simulink library "PTOSim_Lib_org"  (R2014b)
settings: Solver=ode45  StartTime=0.0  StopTime=10.0  RelTol=1e-3
undefined symbols (not defined in the file or in its folder): accum, ddload, gen, machine, motor, pAeq, pAupper_limit, pBeq, pBupper_limit, piston, simu, tot, valve
libraries: PTOSim_Lib x10, WECSim_Lib x2
settings Model: RequirementInfo="{}  %GIDa_42666abb_d6d9_408c_ae24_f6520282b61c"  Creator=sor  LastModifiedBy=rso

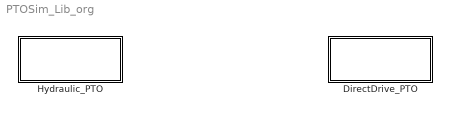
== system PTOSim_Lib_org ==
  DirectDrive_PTO : Subsystem  RequirementInfo="{}  %GIDa_5439fdb4_7c29_433c_8677_23bf92e18f11"
  Hydraulic_PTO : Subsystem  RequirementInfo={} %GIDa_f12a42eb_b9cb_4818_b573_b7dee4183a3b

== system PTOSim_Lib_org/DirectDrive_PTO ==
  Direct Drive PTO : Subsystem  mask{Parameter1=0}
      mask prompts: Parameter1 "pto"
  Electric Machine : Subsystem  RequirementInfo="{}  %GIDa_9a577bd3_d1cd_44c9_a605_4eaf21e33064"  mask{machine=machine}
      mask prompts: machine "Machine Name:"
  Load : Subsystem  mask(PTO-Sim Element){ddload=ddload}
      mask prompts: ddload "Load Name:"

== system PTOSim_Lib_org/Hydraulic_PTO ==
  Accumulator : Subsystem  mask(PTO-Sim Element){accum=accum}
      mask prompts: accum "Accumulator Name:"
  Generator : Subsystem  RequirementInfo="{}  %GIDa_30368e1c_dc2a_4605_bb50_ff3a423f2df5"  mask{gen=gen}
      mask prompts: gen "Generator Name"
  "High Accumulator " : Subsystem  mask(PTO-Sim Element){accum=accum}
      mask prompts: accum "Accumulator Name:"
  Hydraulic PTO : Subsystem  RequirementInfo="{}  %GIDa_b8f519ee_1776_4469_9852_74bfa511eadd"  mask{Parameter1=0}
      mask prompts: Parameter1 "pto"
  Low Accumulator : Subsystem  mask(PTO-Sim Element){accum=accum}
      mask prompts: accum "Accumulator"
  "Motor " : Subsystem  mask{motor=motor}
      mask prompts: motor "Motor Name:"
  "Piston " : Subsystem  RequirementInfo="{}  %GIDa_b30889e8_4129_48f7_be7d_bc9428e6e267"  mask(PTO-Sim Element){piston=piston}
      mask prompts: piston "Piston Name:"
  PistonX : Subsystem  mask{piston=piston}
      mask prompts: piston "Piston X Name:"
  Rectifiying Check Valve : Subsystem  RequirementInfo="{}  %GIDa_a75844df_5079_4f47_95bd_8083cdfec0d7"  mask{valve=valve}
      mask prompts: valve "Valve Name:"

== system PTOSim_Lib_org/DirectDrive_PTO/Direct Drive PTO ==
  vel : Inport
  Electric Machine : PTOSim_Lib/DirectDrive_PTO/Electric Machine  machine=machine
  Load : PTOSim_Lib/DirectDrive_PTO/Load  ddload=ddload
  Terminator1 : Terminator
  force : Outport
  wires:
  Electric Machine/2 -> Load/1
  Load/1 -> Electric Machine/2
  Electric Machine/1 -> force/1
  Load/2 -> Terminator1/1
  vel/1 -> Electric Machine/1

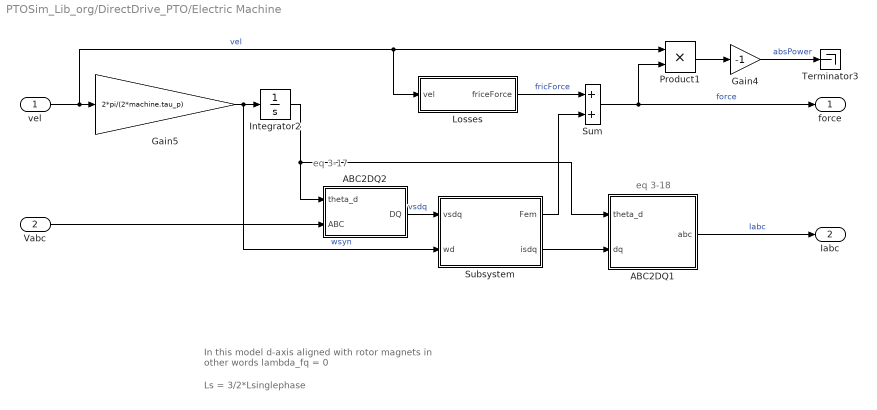
== system PTOSim_Lib_org/DirectDrive_PTO/Electric Machine ==
  note: In this model d-axis aligned with rotor magnets
      | in other words lambda_fq = 0
  note: Ls = 3/2*Lsinglephase
  note: eq 3-17
  note: eq 3-18
  vel : Inport
  Vabc : Inport  Port=2
  ABC2DQ1 : Subsystem
  ABC2DQ2 : Subsystem
  Gain4 : Gain  Gain=-1
  Gain5 : Gain  Gain=2*pi/(2*machine.tau_p)
  Integrator2 : Integrator  InitialCondition=machine.theta_d_0
  Losses : Subsystem
  Product1 : Product
  Subsystem : Subsystem
  Sum : Sum
  Terminator3 : Terminator
  force : Outport
  Iabc : Outport  Port=2
  wires:
  ABC2DQ2/1(DQ) -> Subsystem/1(vsdq)  "vsdq"
  ABC2DQ1/1(abc) -> Iabc/1  "Iabc"
  vel/1 -> Gain5/1, Losses/1(vel), Product1/1  "vel"
  Gain5/1 -> Subsystem/2(wd), Integrator2/1  "wsyn"
  Integrator2/1 -> ABC2DQ2/1(theta_d), ABC2DQ1/1(theta_d)
  Product1/1 -> Gain4/1
  Gain4/1 -> Terminator3/1  "absPower"
  Subsystem/1(Fem) -> Sum/2
  Vabc/1 -> ABC2DQ2/2(ABC)
  Subsystem/2(isdq) -> ABC2DQ1/2(dq)
  Losses/1(friceForce) -> Sum/1  "fricForce"
  Sum/1 -> Product1/2, force/1  "force"

== system PTOSim_Lib_org/DirectDrive_PTO/Load ==
  Iabc : Inport
  Gain : Gain  Gain=-1
  Gain1 : Gain  Gain=ddload.Rload
  Product : Product
  Sum of Elements : Sum  Inputs=+
  Vabc : Outport
  elecPower : Outport  Port=2
  wires:
  Gain/1 -> elecPower/1  "elecPower"
  Gain1/1 -> Product/1, Vabc/1  "Vabc"
  Product/1 -> Sum of Elements/1
  Iabc/1 -> Gain1/1, Product/2
  Sum of Elements/1 -> Gain/1

== system PTOSim_Lib_org/Hydraulic_PTO/Accumulator ==
  volFlowAccum : Inport
  volFlowM : Inport  Port=2
  Constant : Constant
  Constant3 : Constant  Value=accum.pIprecharge
  Constant4 : Constant  Value=accum.VI0
  Divide : Product  Inputs=*/
  Divide1 : Product  Inputs=*/
  Exponent : Constant  Value=1.4
  Integrator4 : Integrator  InitialCondition=accum.VIeq
  Math Function : Math  Operator=pow  SaturateOnIntegerOverflow=on
  Sum : Sum  Inputs=-+
  Sum2 : Sum
  pressure : Outport
  wires:
  Sum2/1 -> Integrator4/1  "volFlowAccum"
  Integrator4/1 -> Divide/1  "volAccum"
  Constant4/1 -> Divide/2
  Constant/1 -> Sum/2
  Divide/1 -> Sum/1
  Exponent/1 -> Math Function/2
  Sum/1 -> Math Function/1
  Math Function/1 -> Divide1/2
  Constant3/1 -> Divide1/1  "pI0"
  Divide1/1 -> pressure/1
  volFlowAccum/1 -> Sum2/1
  volFlowM/1 -> Sum2/2

== system PTOSim_Lib_org/Hydraulic_PTO/Generator ==
  torque : Inport
  omega : Inport  Port=2
  Base Motor Torque : Gain  Gain=-1/gen.TgenBase
  Base Motor Torque1 : Gain  Gain=1/gen.omegaBase
  Base Motor Torque2 : Gain  Gain=gen.driveEff
  Base Motor Torque3 : Gain  Gain=1/100
  PM p.u. Efficiency Lookup Table : Lookup_n-D  BreakpointsForDimension1=tot.Tpu(:,1)  BreakpointsForDimension2=tot.omegapu(1,:)  Table=tot.eff  InterpMethod=Flat  InputSameDT=on
  Product : Product  RndMeth=Zero
  Product1 : Product  RndMeth=Zero
  elecPower : Outport
  wires:
  Base Motor Torque2/1 -> elecPower/1  "elecPower"
  Product1/1 -> Base Motor Torque2/1
  Product/1 -> Product1/1  "genPower"
  Base Motor Torque3/1 -> Product1/2  "genEff"
  PM p.u. Efficiency Lookup Table/1 -> Base Motor Torque3/1
  omega/1 -> Product/2, Base Motor Torque1/1
  Base Motor Torque1/1 -> PM p.u. Efficiency Lookup Table/2  "omegaPU"
  torque/1 -> Base Motor Torque/1, Product/1
  Base Motor Torque/1 -> PM p.u. Efficiency Lookup Table/1  "torquePU"

== system PTOSim_Lib_org/Hydraulic_PTO/High Accumulator  ==
  volFlowHigh : Inport
  volFlowM : Inport  Port=2
  Constant : Constant
  Constant3 : Constant  Value=accum.pCprecharge
  Constant4 : Constant  Value=accum.VC0
  Divide : Product  Inputs=*/
  Divide1 : Product  Inputs=*/
  Exponent : Constant  Value=1.4
  Integrator4 : Integrator  InitialCondition=accum.VCeq
  Math Function : Math  Operator=pow  SaturateOnIntegerOverflow=on
  Sum : Sum  Inputs=-+
  Sum2 : Sum
  pressure : Outport
  wires:
  Sum2/1 -> Integrator4/1  "volFlowC"
  Integrator4/1 -> Divide/1  "volC"
  Constant4/1 -> Divide/2
  Constant/1 -> Sum/2
  Divide/1 -> Sum/1
  Exponent/1 -> Math Function/2
  Sum/1 -> Math Function/1
  Math Function/1 -> Divide1/2
  Constant3/1 -> Divide1/1  "pC0"
  Divide1/1 -> pressure/1
  volFlowHigh/1 -> Sum2/1
  volFlowM/1 -> Sum2/2

== system PTOSim_Lib_org/Hydraulic_PTO/Hydraulic PTO ==
  pos : Inport
  vel : Inport  Port=2
  Accumulator : PTOSim_Lib/Hydraulic_PTO/Accumulator  accum=highAccum
  Accumulator1 : PTOSim_Lib/Hydraulic_PTO/Accumulator  accum=lowAccum
  Generator : PTOSim_Lib/Hydraulic_PTO/Generator  gen=gen
  "Motor " : PTOSim_Lib/Hydraulic_PTO/Motor   motor=motor
  "Piston " : PTOSim_Lib/Hydraulic_PTO/Piston    piston=piston
  Rectifiying Check Valve : PTOSim_Lib/Hydraulic_PTO/Rectifiying  Check Valve  valve=valve
  Terminator : Terminator
  force : Outport
  wires:
  pos/1 -> "Piston "/1  "pos"
  vel/1 -> "Piston "/2  "vel"
  "Piston "/2 -> Rectifiying Check Valve/1  "topPressure"
  "Piston "/3 -> Rectifiying Check Valve/2  "bottomPressure"
  "Motor "/1 -> Generator/1
  "Motor "/2 -> Generator/2
  Accumulator/1 -> "Motor "/1, Rectifiying Check Valve/3  "highPressure"
  Accumulator1/1 -> Rectifiying Check Valve/4, "Motor "/2  "lowPressure"
  Generator/1 -> Terminator/1
  "Piston "/1 -> force/1
  Rectifiying Check Valve/1 -> "Piston "/3
  Rectifiying Check Valve/2 -> "Piston "/4
  Rectifiying Check Valve/3 -> Accumulator/1
  Rectifiying Check Valve/4 -> Accumulator1/1
  "Motor "/4 -> Accumulator1/2
  "Motor "/3 -> Accumulator/2

== system PTOSim_Lib_org/Hydraulic_PTO/Low Accumulator ==
  volFlowLow : Inport
  volFlowM : Inport  Port=2
  Constant : Constant
  Constant3 : Constant  Value=accum.pDprecharge
  Constant4 : Constant  Value=accum.VD0
  Divide : Product  Inputs=*/
  Divide1 : Product  Inputs=*/
  Exponent : Constant  Value=1.4
  Integrator4 : Integrator  InitialCondition=accum.VDeq
  Math Function : Math  Operator=pow  SaturateOnIntegerOverflow=on
  Sum : Sum  Inputs=-+
  Sum2 : Sum
  pressure : Outport
  wires:
  Sum2/1 -> Integrator4/1  "volFlowD"
  Integrator4/1 -> Divide/1  "volD"
  Constant4/1 -> Divide/2
  Constant/1 -> Sum/2
  Divide/1 -> Sum/1
  Exponent/1 -> Math Function/2
  Sum/1 -> Math Function/1
  Math Function/1 -> Divide1/2
  Constant3/1 -> Divide1/1  "pD0"
  Divide1/1 -> pressure/1
  volFlowLow/1 -> Sum2/1
  volFlowM/1 -> Sum2/2

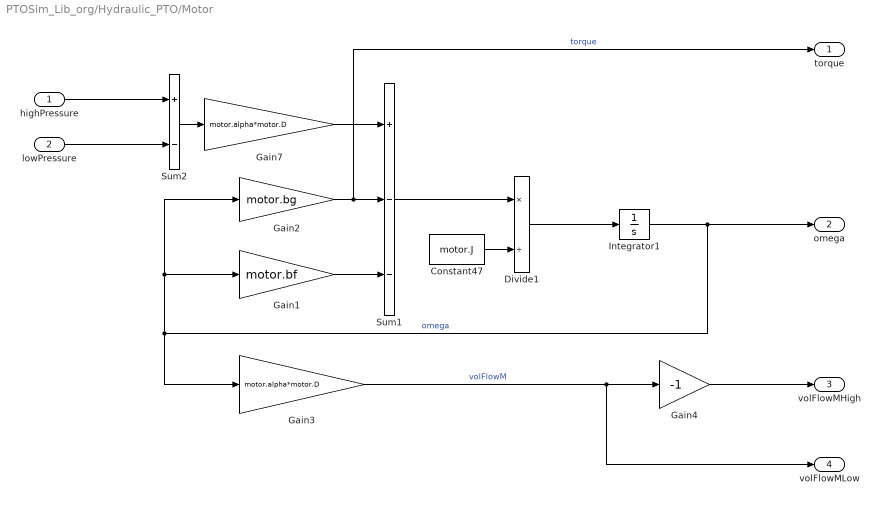
== system PTOSim_Lib_org/Hydraulic_PTO/Motor  ==
  highPressure : Inport
  lowPressure : Inport  Port=2
  Constant47 : Constant  Value=motor.J
  Divide1 : Product  Inputs=*/
  Gain1 : Gain  Gain=motor.bf
  Gain2 : Gain  Gain=motor.bg
  Gain3 : Gain  Gain=motor.alpha*motor.D
  Gain4 : Gain  Gain=-1
  Gain7 : Gain  Gain=motor.alpha*motor.D
  Integrator1 : Integrator  InitialCondition=motor.omegaInit
  Sum1 : Sum  Inputs=+--
  Sum2 : Sum  Inputs=+-
  torque : Outport
  omega : Outport  Port=2
  volFlowMHigh : Outport  Port=3
  volFlowMLow : Outport  Port=4
  wires:
  Gain7/1 -> Sum1/1
  Gain2/1 -> torque/1, Sum1/2  "torque"
  Gain1/1 -> Sum1/3
  Sum1/1 -> Divide1/1
  Constant47/1 -> Divide1/2
  Divide1/1 -> Integrator1/1
  Integrator1/1 -> omega/1, Gain3/1, Gain2/1, Gain1/1  "omega"
  Gain3/1 -> volFlowMLow/1, Gain4/1  "volFlowM"
  highPressure/1 -> Sum2/1
  lowPressure/1 -> Sum2/2
  Sum2/1 -> Gain7/1
  Gain4/1 -> volFlowMHigh/1

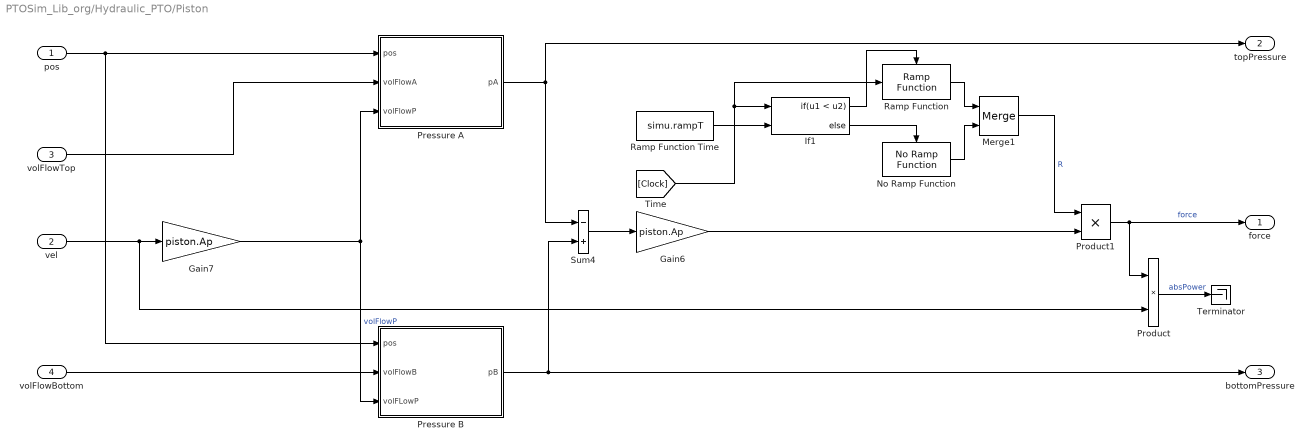
== system PTOSim_Lib_org/Hydraulic_PTO/Piston  ==
  pos : Inport
  vel : Inport  Port=2
  volFlowTop : Inport  Port=3
  volFlowBottom : Inport  Port=4
  Gain6 : Gain  Gain=piston.Ap
  Gain7 : Gain  Gain=piston.Ap
  If1 : If  NumInputs=2  IfExpression=u1 < u2
  Merge1 : Merge
  No Ramp Function : WECSim_Lib/Body Elements/Rigid Body/Wave Diffraction and Excitation Force Calculation/No Ramp Function
  Pressure A : Subsystem
  Pressure B : Subsystem  RequirementInfo="{}  %GIDa_18ee15fe_6148_4b69_b054_be19d4b47378"
  Product : Product
  Product1 : Product
  Ramp Function : WECSim_Lib/Body Elements/Rigid Body/Wave Diffraction and Excitation Force Calculation/Ramp Function
  Ramp Function Time : Constant  Value=simu.rampT
  Sum4 : Sum  Inputs=-+
  Terminator : Terminator
  force : Outport
  topPressure : Outport  Port=2
  bottomPressure : Outport  Port=3
  wires:
  Pressure A/1(pA) -> Sum4/1, topPressure/1
  Pressure B/1(pB) -> Sum4/2, bottomPressure/1
  Gain7/1 -> Pressure B/3(volFLowP), Pressure A/3(volFlowP)  "volFlowP"
  Product/1 -> Terminator/1  "absPower"
  pos/1 -> Pressure B/1(pos), Pressure A/1(pos)
  vel/1 -> Product/2, Gain7/1
  Sum4/1 -> Gain6/1
  [Clock] -> If1/1, Ramp Function/1
  Merge1/1 -> Product1/1  "R"
  Ramp Function Time/1 -> If1/2
  If1/2 -> No Ramp Function/Action
  If1/1 -> Ramp Function/Action
  Ramp Function/1 -> Merge1/1
  No Ramp Function/1 -> Merge1/2
  Gain6/1 -> Product1/2
  Product1/1 -> force/1, Product/1  "force"
  volFlowTop/1 -> Pressure A/2(volFlowA)
  volFlowBottom/1 -> Pressure B/2(volFlowB)

== system PTOSim_Lib_org/Hydraulic_PTO/PistonX ==
  pos : Inport
  vel : Inport  Port=2
  volFlowTop : Inport  Port=3
  volFlowBottom : Inport  Port=4
  Gain6 : Gain  Gain=piston.Ap
  Gain7 : Gain  Gain=piston.Ap
  Pressure A : PTOSim_Lib/Hydraulic_PTO/Piston  /Pressure A
  Pressure B : PTOSim_Lib/Hydraulic_PTO/Piston  /Pressure B
  Product : Product
  Sum4 : Sum  Inputs=-+
  Terminator : Terminator
  force : Outport
  topPressure : Outport  Port=2
  bottomPressure : Outport  Port=3
  wires:
  Pressure A/1 -> Sum4/1, topPressure/1
  Pressure B/1 -> Sum4/2, bottomPressure/1
  Gain7/1 -> Pressure B/3, Pressure A/3  "volFlowP"
  Product/1 -> Terminator/1  "absPower"
  pos/1 -> Pressure B/1, Pressure A/1
  vel/1 -> Product/2, Gain7/1
  Sum4/1 -> Gain6/1
  Gain6/1 -> force/1, Product/1  "force"
  volFlowTop/1 -> Pressure A/2
  volFlowBottom/1 -> Pressure B/2

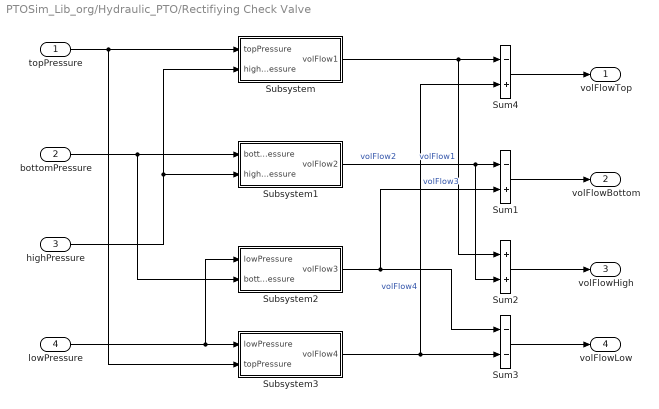
== system PTOSim_Lib_org/Hydraulic_PTO/Rectifiying Check Valve ==
  topPressure : Inport
  bottomPressure : Inport  Port=2
  highPressure : Inport  Port=3
  lowPressure : Inport  Port=4
  Subsystem : Subsystem  RequirementInfo="{}  %GIDa_43e7490a_26e5_4c96_a755_05599e7ab58d"
  Subsystem1 : Subsystem
  Subsystem2 : Subsystem
  Subsystem3 : Subsystem  RequirementInfo="{}  %GIDa_1d14c02d_1c58_4958_a821_20fe782ea22d"
  Sum1 : Sum  Inputs=-+
  Sum2 : Sum
  Sum3 : Sum  Inputs=--
  Sum4 : Sum  Inputs=-+
  volFlowTop : Outport
  volFlowBottom : Outport  Port=2
  volFlowHigh : Outport  Port=3
  volFlowLow : Outport  Port=4
  wires:
  topPressure/1 -> Subsystem3/2(topPressure), Subsystem/1(topPressure)
  bottomPressure/1 -> Subsystem2/2(bottomPressure), Subsystem1/1(bottomPressure)
  highPressure/1 -> Subsystem1/2(highPressure), Subsystem/2(highPressure)
  lowPressure/1 -> Subsystem2/1(lowPressure), Subsystem3/1(lowPressure)
  Subsystem3/1(volFlow4) -> Sum4/2, Sum3/2  "volFlow4"
  Subsystem2/1(volFlow3) -> Sum3/1, Sum1/2  "volFlow3"
  Subsystem1/1(volFlow2) -> Sum2/2, Sum1/1  "volFlow2"
  Subsystem/1(volFlow1) -> Sum2/1, Sum4/1  "volFlow1"
  Sum4/1 -> volFlowTop/1
  Sum1/1 -> volFlowBottom/1
  Sum2/1 -> volFlowHigh/1
  Sum3/1 -> volFlowLow/1

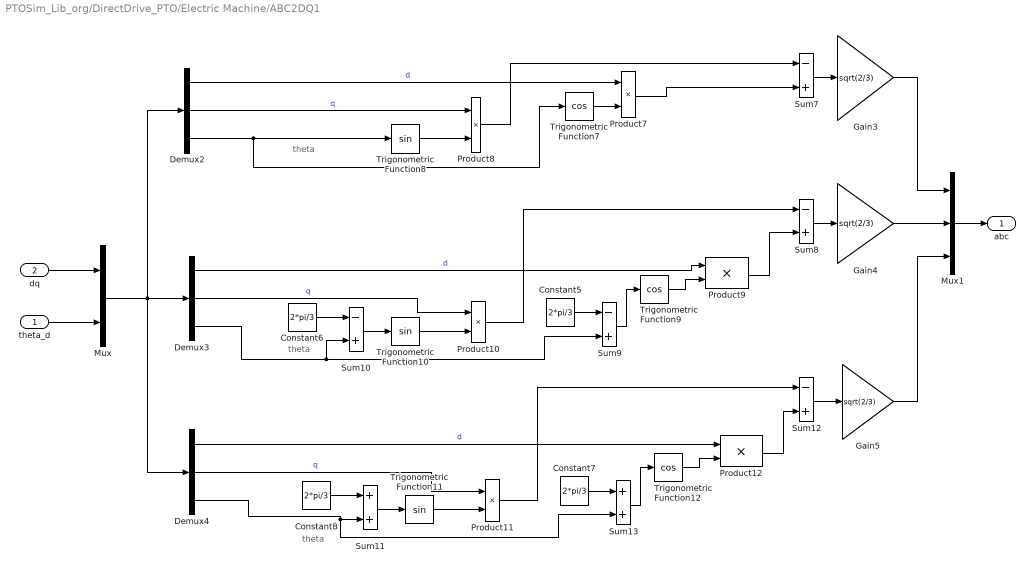
== system PTOSim_Lib_org/DirectDrive_PTO/Electric Machine/ABC2DQ1 ==
  note: theta
  note: theta
  note: theta
  theta_d : Inport
  dq : Inport  Port=2
  Constant{5..8} (4 alike) : Constant  Value=2*pi/3
  Demux2 : Demux  Outputs=3
  Demux3 : Demux  Outputs=3
  Demux4 : Demux  Outputs=3
  Gain3 : Gain  Gain=sqrt(2/3)  SaturateOnIntegerOverflow=on  OutDataTypeStr=Inherit: Same as input  ParamDataTypeStr=Inherit: Same as input
  Gain4 : Gain  Gain=sqrt(2/3)  SaturateOnIntegerOverflow=on  OutDataTypeStr=Inherit: Same as input  ParamDataTypeStr=Inherit: Same as input
  Gain5 : Gain  Gain=sqrt(2/3)  SaturateOnIntegerOverflow=on  OutDataTypeStr=Inherit: Same as input  ParamDataTypeStr=Inherit: Same as input
  Mux : Mux  Inputs=2
  Mux1 : Mux  Inputs=3
  Product{7..12} (6 alike) : Product  SaturateOnIntegerOverflow=on  InputSameDT=on  OutDataTypeStr=Inherit: Same as first input
  Sum{7..10,12} (5 alike) : Sum  Inputs=-+  SaturateOnIntegerOverflow=on  InputSameDT=on  OutDataTypeStr=Inherit: Same as first input
  Sum11 : Sum  SaturateOnIntegerOverflow=on  InputSameDT=on  OutDataTypeStr=Inherit: Same as first input
  Sum13 : Sum  SaturateOnIntegerOverflow=on  InputSameDT=on  OutDataTypeStr=Inherit: Same as first input
  Trigonometric Function10 : Trigonometry
  Trigonometric Function11 : Trigonometry
  Trigonometric Function12 : Trigonometry  Operator=cos
  Trigonometric Function7 : Trigonometry  Operator=cos
  Trigonometric Function8 : Trigonometry
  Trigonometric Function9 : Trigonometry  Operator=cos
  abc : Outport
  wires:
  Mux1/1 -> abc/1
  dq/1 -> Mux/1
  theta_d/1 -> Mux/2
  Mux/1 -> Demux4/1, Demux2/1, Demux3/1
  Trigonometric Function7/1 -> Product7/2
  Demux2/1 -> Product7/1  "d"
  Product7/1 -> Sum7/2
  Product8/1 -> Sum7/1
  Demux2/3 -> Trigonometric Function8/1, Trigonometric Function7/1
  Demux2/2 -> Product8/1  "q"
  Trigonometric Function9/1 -> Product9/2
  Demux3/1 -> Product9/1  "d"
  Product9/1 -> Sum8/2
  Product10/1 -> Sum8/1
  Demux3/3 -> Sum10/2, Sum9/2
  Trigonometric Function10/1 -> Product10/2
  Demux3/2 -> Product10/1  "q"
  Sum9/1 -> Trigonometric Function9/1
  Constant5/1 -> Sum9/1
  Sum10/1 -> Trigonometric Function10/1
  Constant6/1 -> Sum10/1
  Trigonometric Function12/1 -> Product12/2
  Demux4/1 -> Product12/1  "d"
  Product12/1 -> Sum12/2
  Product11/1 -> Sum12/1
  Demux4/3 -> Sum13/2, Sum11/2
  Trigonometric Function11/1 -> Product11/2
  Demux4/2 -> Product11/1  "q"
  Sum13/1 -> Trigonometric Function12/1
  Constant7/1 -> Sum13/1
  Sum11/1 -> Trigonometric Function11/1
  Constant8/1 -> Sum11/1
  Sum7/1 -> Gain3/1
  Sum8/1 -> Gain4/1
  Sum12/1 -> Gain5/1
  Gain3/1 -> Mux1/1
  Gain4/1 -> Mux1/2
  Gain5/1 -> Mux1/3
  Trigonometric Function8/1 -> Product8/2

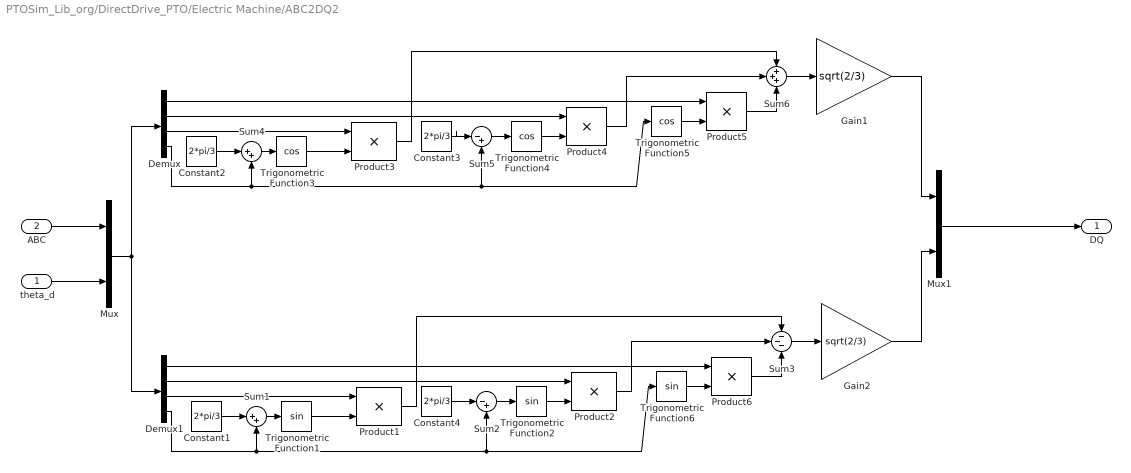
== system PTOSim_Lib_org/DirectDrive_PTO/Electric Machine/ABC2DQ2 ==
  theta_d : Inport
  ABC : Inport  Port=2
  Constant{1..4} (4 alike) : Constant  Value=2*pi/3
  Demux : Demux
  Demux1 : Demux
  Gain1 : Gain  Gain=sqrt(2/3)  SaturateOnIntegerOverflow=on  OutDataTypeStr=Inherit: Same as input  ParamDataTypeStr=Inherit: Same as input
  Gain2 : Gain  Gain=sqrt(2/3)  SaturateOnIntegerOverflow=on  OutDataTypeStr=Inherit: Same as input  ParamDataTypeStr=Inherit: Same as input
  Mux : Mux  Inputs=2
  Mux1 : Mux  Inputs=2
  Product{1..6} (6 alike) : Product  SaturateOnIntegerOverflow=on  InputSameDT=on  OutDataTypeStr=Inherit: Same as first input
  Sum1 : Sum  Inputs=|++  SaturateOnIntegerOverflow=on  InputSameDT=on  OutDataTypeStr=Inherit: Same as first input
  Sum2 : Sum  Inputs=|-+  SaturateOnIntegerOverflow=on  InputSameDT=on  OutDataTypeStr=Inherit: Same as first input
  Sum3 : Sum  Inputs=---  SaturateOnIntegerOverflow=on  InputSameDT=on  OutDataTypeStr=Inherit: Same as first input
  Sum4 : Sum  Inputs=|++  SaturateOnIntegerOverflow=on  InputSameDT=on  OutDataTypeStr=Inherit: Same as first input
  Sum5 : Sum  Inputs=|-+  SaturateOnIntegerOverflow=on  InputSameDT=on  OutDataTypeStr=Inherit: Same as first input
  Sum6 : Sum  Inputs=+++  SaturateOnIntegerOverflow=on  InputSameDT=on  OutDataTypeStr=Inherit: Same as first input
  Trigonometric Function1 : Trigonometry
  Trigonometric Function2 : Trigonometry
  Trigonometric Function3 : Trigonometry  Operator=cos
  Trigonometric Function4 : Trigonometry  Operator=cos
  Trigonometric Function5 : Trigonometry  Operator=cos
  Trigonometric Function6 : Trigonometry
  DQ : Outport
  wires:
  Mux1/1 -> DQ/1
  Product5/1 -> Sum6/3
  Constant2/1 -> Sum4/1
  Sum5/1 -> Trigonometric Function4/1
  Trigonometric Function4/1 -> Product4/2
  Trigonometric Function5/1 -> Product5/2
  Constant3/1 -> Sum5/1
  Sum6/1 -> Gain1/1
  Product3/1 -> Sum6/1
  Product4/1 -> Sum6/2
  Trigonometric Function3/1 -> Product3/2
  Gain1/1 -> Mux1/1
  ABC/1 -> Mux/1
  theta_d/1 -> Mux/2
  Demux/1 -> Product5/1
  Demux/2 -> Product4/1
  Demux/3 -> Product3/1
  Demux/4 -> Sum5/2, Trigonometric Function5/1, Sum4/2
  Mux/1 -> Demux/1, Demux1/1
  Sum4/1 -> Trigonometric Function3/1
  Product6/1 -> Sum3/3
  Constant1/1 -> Sum1/1
  Sum2/1 -> Trigonometric Function2/1
  Trigonometric Function2/1 -> Product2/2
  Trigonometric Function6/1 -> Product6/2
  Constant4/1 -> Sum2/1
  Sum3/1 -> Gain2/1
  Product1/1 -> Sum3/1
  Product2/1 -> Sum3/2
  Trigonometric Function1/1 -> Product1/2
  Gain2/1 -> Mux1/2
  Demux1/1 -> Product6/1
  Demux1/2 -> Product2/1
  Demux1/3 -> Product1/1
  Demux1/4 -> Sum1/2, Trigonometric Function6/1, Sum2/2
  Sum1/1 -> Trigonometric Function1/1

== system PTOSim_Lib_org/DirectDrive_PTO/Electric Machine/Losses ==
  vel : Inport
  Gain : Gain  Gain=machine.Bfric
  friceForce : Outport
  wires:
  vel/1 -> Gain/1
  Gain/1 -> friceForce/1

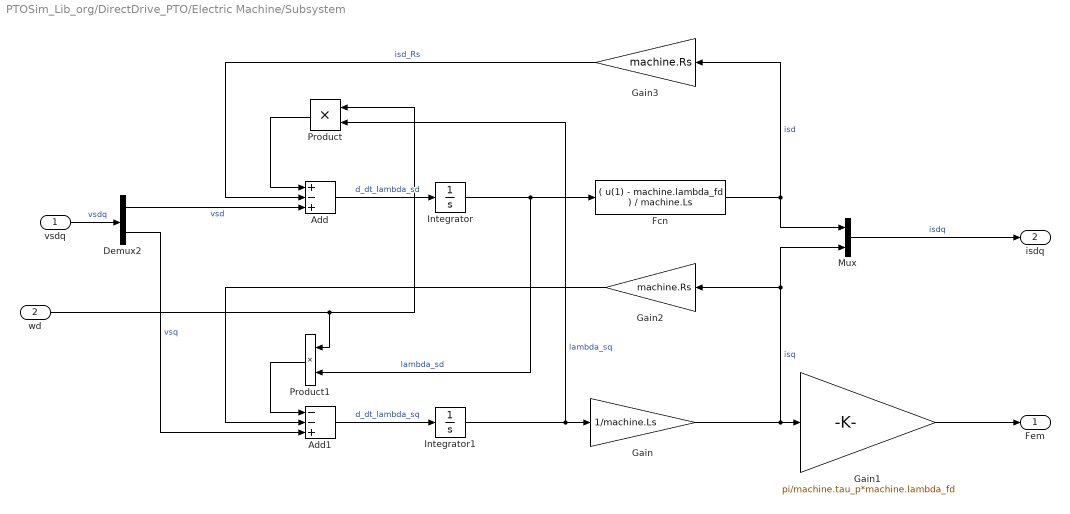
== system PTOSim_Lib_org/DirectDrive_PTO/Electric Machine/Subsystem ==
  vsdq : Inport
  wd : Inport  Port=2
  Add : Sum  Inputs=+-+
  Add1 : Sum  Inputs=--+
  Demux2 : Demux  Outputs=2
  Fcn : Fcn  Expr=( u(1) - machine.lambda_fd ) / machine.Ls
  Gain : Gain  Gain=1/machine.Ls
  Gain1 : Gain  Gain=pi/machine.tau_p*machine.lambda_fd
  Gain2 : Gain  Gain=machine.Rs
  Gain3 : Gain  Gain=machine.Rs
  Integrator : Integrator  InitialCondition=machine.lambda_sd_0
  Integrator1 : Integrator  InitialCondition=machine.lambda_sq_0
  Mux : Mux  Inputs=2
  Product : Product  RndMeth=Zero
  Product1 : Product  RndMeth=Zero
  Fem : Outport
  isdq : Outport  Port=2
  wires:
  Add/1 -> Integrator/1  "d_dt_lambda_sd"
  Integrator/1 -> Product1/2, Fcn/1  "lambda_sd"
  Fcn/1 -> Gain3/1, Mux/1  "isd"
  Product/1 -> Add/1
  Add1/1 -> Integrator1/1  "d_dt_lambda_sq"
  Integrator1/1 -> Gain/1, Product/2  "lambda_sq"
  wd/1 -> Product1/1, Product/1
  Gain/1 -> Gain1/1, Gain2/1, Mux/2  "isq"
  Product1/1 -> Add1/1
  Demux2/1 -> Add/3  "vsd"
  Demux2/2 -> Add1/3  "vsq"
  vsdq/1 -> Demux2/1  "vsdq"
  Gain3/1 -> Add/2  "isd_Rs"
  Gain2/1 -> Add1/2
  Mux/1 -> isdq/1  "isdq"
  Gain1/1 -> Fem/1

== system PTOSim_Lib_org/Hydraulic_PTO/Piston /Pressure A ==
  pos : Inport
  volFlowA : Inport  Port=2
  volFlowP : Inport  Port=3
  Constant : Constant  Value=piston.Vo
  Divide : Product  Inputs=*/
  Gain1 : Gain  Gain=piston.Beta_e
  Gain2 : Gain  Gain=piston.Ap
  Integrator2 : Integrator  InitialCondition=piston.pAi  UpperSaturationLimit=pAupper_limit  LowerSaturationLimit=pAeq
  Sum : Sum
  Sum1 : Sum  Inputs=-+
  pA : Outport
  wires:
  Sum/1 -> Gain1/1
  pos/1 -> Gain2/1
  Gain2/1 -> Sum1/1
  Constant/1 -> Sum1/2
  Gain1/1 -> Divide/1
  Sum1/1 -> Divide/2
  volFlowA/1 -> Sum/1
  Divide/1 -> Integrator2/1  "pAdot"
  Integrator2/1 -> pA/1
  volFlowP/1 -> Sum/2

== system PTOSim_Lib_org/Hydraulic_PTO/Piston /Pressure B ==
  pos : Inport
  volFlowB : Inport  Port=2
  volFLowP : Inport  Port=3
  Constant1 : Constant  Value=piston.Vo
  Divide1 : Product  Inputs=*/
  Gain4 : Gain  Gain=piston.Beta_e
  Gain5 : Gain  Gain=piston.Ap
  Integrator3 : Integrator  InitialCondition=piston.pBi  UpperSaturationLimit=pBupper_limit  LowerSaturationLimit=pBeq
  Sum2 : Sum  Inputs=+-
  Sum3 : Sum
  pB : Outport
  wires:
  Sum2/1 -> Gain4/1
  pos/1 -> Gain5/1
  Gain5/1 -> Sum3/1
  Constant1/1 -> Sum3/2
  Gain4/1 -> Divide1/1
  Sum3/1 -> Divide1/2
  Divide1/1 -> Integrator3/1  "pBdot"
  volFlowB/1 -> Sum2/1
  Integrator3/1 -> pB/1
  volFLowP/1 -> Sum2/2

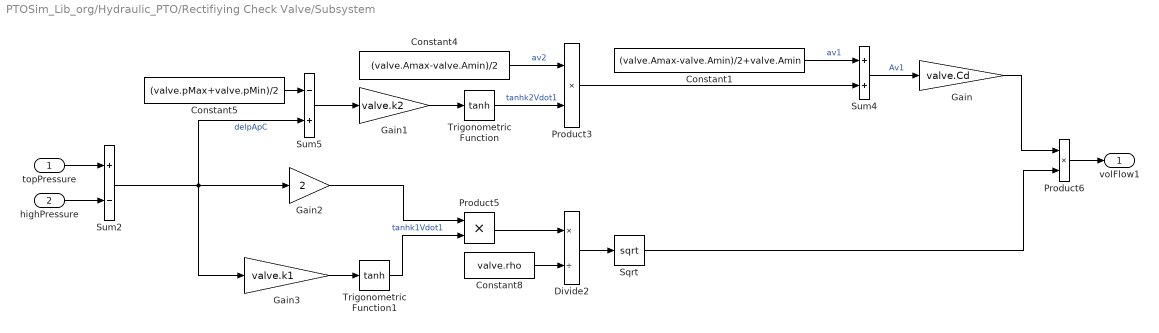
== system PTOSim_Lib_org/Hydraulic_PTO/Rectifiying Check Valve/Subsystem ==
  topPressure : Inport
  highPressure : Inport  Port=2
  Constant1 : Constant  Value=(valve.Amax-valve.Amin)/2+valve.Amin
  Constant4 : Constant  Value=(valve.Amax-valve.Amin)/2
  Constant5 : Constant  Value=(valve.pMax+valve.pMin)/2
  Constant8 : Constant  Value=valve.rho
  Divide2 : Product  Inputs=*/
  Gain : Gain  Gain=valve.Cd
  Gain1 : Gain  Gain=valve.k2
  Gain2 : Gain  Gain=2
  Gain3 : Gain  Gain=valve.k1
  Product3 : Product
  Product5 : Product
  Product6 : Product
  Sqrt : Sqrt  SaturateOnIntegerOverflow=on
  Sum2 : Sum  Inputs=+-
  Sum4 : Sum
  Sum5 : Sum  Inputs=-+
  Trigonometric Function : Trigonometry  Operator=tanh
  Trigonometric Function1 : Trigonometry  Operator=tanh
  volFlow1 : Outport
  wires:
  Gain1/1 -> Trigonometric Function/1
  Trigonometric Function/1 -> Product3/2  "tanhk2Vdot1"
  Product3/1 -> Sum4/2
  Sum5/1 -> Gain1/1
  Sum4/1 -> Gain/1  "Av1"
  Gain3/1 -> Trigonometric Function1/1
  Gain2/1 -> Product5/1
  Trigonometric Function1/1 -> Product5/2  "tanhk1Vdot1"
  Sqrt/1 -> Product6/2
  Gain/1 -> Product6/1
  Constant8/1 -> Divide2/2
  Product5/1 -> Divide2/1
  Divide2/1 -> Sqrt/1
  topPressure/1 -> Sum2/1
  highPressure/1 -> Sum2/2
  Product6/1 -> volFlow1/1
  Constant4/1 -> Product3/1  "av2"
  Constant5/1 -> Sum5/1
  Constant1/1 -> Sum4/1  "av1"
  Sum2/1 -> Gain3/1, Sum5/2, Gain2/1  "delpApC"

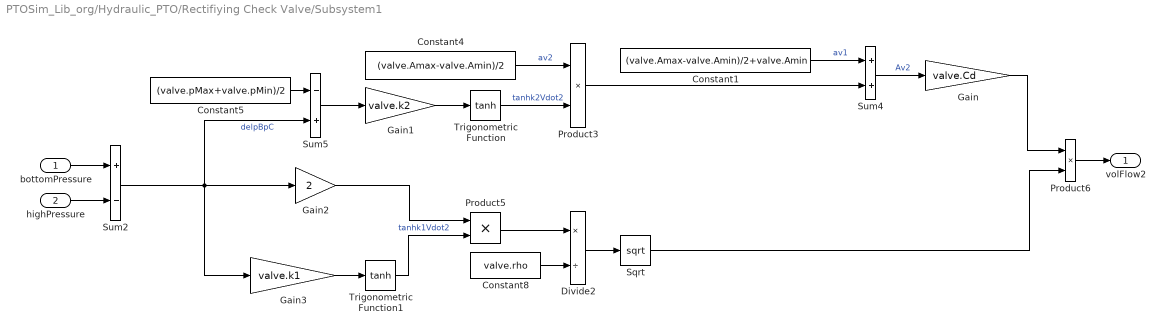
== system PTOSim_Lib_org/Hydraulic_PTO/Rectifiying Check Valve/Subsystem1 ==
  bottomPressure : Inport
  highPressure : Inport  Port=2
  Constant1 : Constant  Value=(valve.Amax-valve.Amin)/2+valve.Amin
  Constant4 : Constant  Value=(valve.Amax-valve.Amin)/2
  Constant5 : Constant  Value=(valve.pMax+valve.pMin)/2
  Constant8 : Constant  Value=valve.rho
  Divide2 : Product  Inputs=*/
  Gain : Gain  Gain=valve.Cd
  Gain1 : Gain  Gain=valve.k2
  Gain2 : Gain  Gain=2
  Gain3 : Gain  Gain=valve.k1
  Product3 : Product
  Product5 : Product
  Product6 : Product
  Sqrt : Sqrt  SaturateOnIntegerOverflow=on
  Sum2 : Sum  Inputs=+-
  Sum4 : Sum
  Sum5 : Sum  Inputs=-+
  Trigonometric Function : Trigonometry  Operator=tanh
  Trigonometric Function1 : Trigonometry  Operator=tanh
  volFlow2 : Outport
  wires:
  Gain1/1 -> Trigonometric Function/1
  Trigonometric Function/1 -> Product3/2  "tanhk2Vdot2"
  Product3/1 -> Sum4/2
  Sum5/1 -> Gain1/1
  Sum4/1 -> Gain/1  "Av2"
  Gain3/1 -> Trigonometric Function1/1
  Gain2/1 -> Product5/1
  Trigonometric Function1/1 -> Product5/2  "tanhk1Vdot2"
  Sqrt/1 -> Product6/2
  Gain/1 -> Product6/1
  Constant8/1 -> Divide2/2
  Product5/1 -> Divide2/1
  Divide2/1 -> Sqrt/1
  bottomPressure/1 -> Sum2/1
  highPressure/1 -> Sum2/2
  Product6/1 -> volFlow2/1
  Constant4/1 -> Product3/1  "av2"
  Constant5/1 -> Sum5/1
  Constant1/1 -> Sum4/1  "av1"
  Sum2/1 -> Gain3/1, Sum5/2, Gain2/1  "delpBpC"

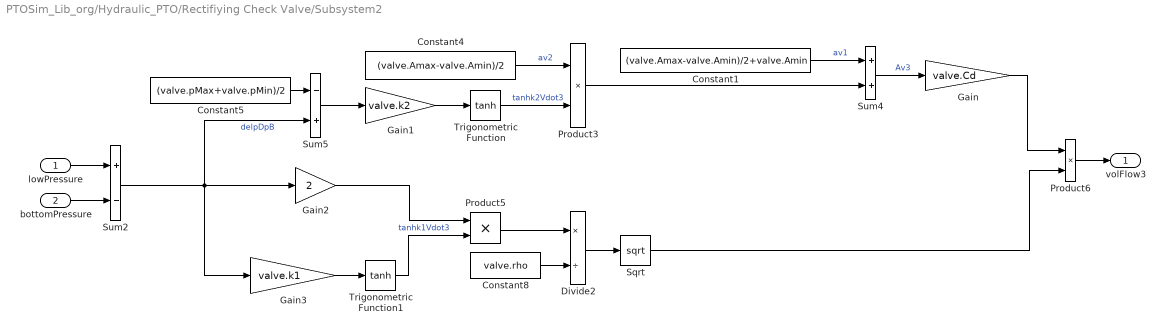
== system PTOSim_Lib_org/Hydraulic_PTO/Rectifiying Check Valve/Subsystem2 ==
  lowPressure : Inport
  bottomPressure : Inport  Port=2
  Constant1 : Constant  Value=(valve.Amax-valve.Amin)/2+valve.Amin
  Constant4 : Constant  Value=(valve.Amax-valve.Amin)/2
  Constant5 : Constant  Value=(valve.pMax+valve.pMin)/2
  Constant8 : Constant  Value=valve.rho
  Divide2 : Product  Inputs=*/
  Gain : Gain  Gain=valve.Cd
  Gain1 : Gain  Gain=valve.k2
  Gain2 : Gain  Gain=2
  Gain3 : Gain  Gain=valve.k1
  Product3 : Product
  Product5 : Product
  Product6 : Product
  Sqrt : Sqrt  SaturateOnIntegerOverflow=on
  Sum2 : Sum  Inputs=+-
  Sum4 : Sum
  Sum5 : Sum  Inputs=-+
  Trigonometric Function : Trigonometry  Operator=tanh
  Trigonometric Function1 : Trigonometry  Operator=tanh
  volFlow3 : Outport
  wires:
  Gain1/1 -> Trigonometric Function/1
  Trigonometric Function/1 -> Product3/2  "tanhk2Vdot3"
  Product3/1 -> Sum4/2
  Sum5/1 -> Gain1/1
  Sum4/1 -> Gain/1  "Av3"
  Gain3/1 -> Trigonometric Function1/1
  Gain2/1 -> Product5/1
  Trigonometric Function1/1 -> Product5/2  "tanhk1Vdot3"
  Sqrt/1 -> Product6/2
  Gain/1 -> Product6/1
  Constant8/1 -> Divide2/2
  Product5/1 -> Divide2/1
  Divide2/1 -> Sqrt/1
  lowPressure/1 -> Sum2/1
  bottomPressure/1 -> Sum2/2
  Product6/1 -> volFlow3/1
  Constant4/1 -> Product3/1  "av2"
  Constant5/1 -> Sum5/1
  Constant1/1 -> Sum4/1  "av1"
  Sum2/1 -> Gain3/1, Sum5/2, Gain2/1  "delpDpB"

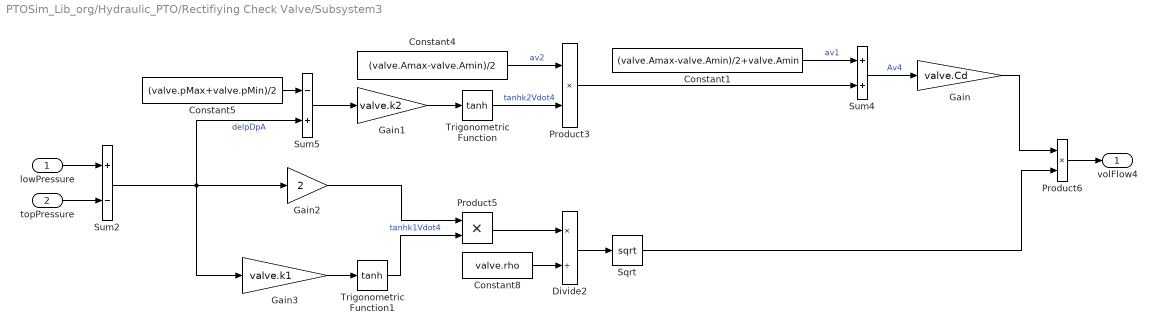
== system PTOSim_Lib_org/Hydraulic_PTO/Rectifiying Check Valve/Subsystem3 ==
  lowPressure : Inport
  topPressure : Inport  Port=2
  Constant1 : Constant  Value=(valve.Amax-valve.Amin)/2+valve.Amin
  Constant4 : Constant  Value=(valve.Amax-valve.Amin)/2
  Constant5 : Constant  Value=(valve.pMax+valve.pMin)/2
  Constant8 : Constant  Value=valve.rho
  Divide2 : Product  Inputs=*/
  Gain : Gain  Gain=valve.Cd
  Gain1 : Gain  Gain=valve.k2
  Gain2 : Gain  Gain=2
  Gain3 : Gain  Gain=valve.k1
  Product3 : Product
  Product5 : Product
  Product6 : Product
  Sqrt : Sqrt  SaturateOnIntegerOverflow=on
  Sum2 : Sum  Inputs=+-
  Sum4 : Sum
  Sum5 : Sum  Inputs=-+
  Trigonometric Function : Trigonometry  Operator=tanh
  Trigonometric Function1 : Trigonometry  Operator=tanh
  volFlow4 : Outport
  wires:
  Gain1/1 -> Trigonometric Function/1
  Trigonometric Function/1 -> Product3/2  "tanhk2Vdot4"
  Product3/1 -> Sum4/2
  Sum5/1 -> Gain1/1
  Sum4/1 -> Gain/1  "Av4"
  Gain3/1 -> Trigonometric Function1/1
  Gain2/1 -> Product5/1
  Trigonometric Function1/1 -> Product5/2  "tanhk1Vdot4"
  Sqrt/1 -> Product6/2
  Gain/1 -> Product6/1
  Constant8/1 -> Divide2/2
  Product5/1 -> Divide2/1
  Divide2/1 -> Sqrt/1
  lowPressure/1 -> Sum2/1
  topPressure/1 -> Sum2/2
  Product6/1 -> volFlow4/1
  Constant4/1 -> Product3/1  "av2"
  Constant5/1 -> Sum5/1
  Constant1/1 -> Sum4/1  "av1"
  Sum2/1 -> Gain3/1, Sum5/2, Gain2/1  "delpDpA"
